simulink model "Solar_Panel_Tutorial"  (R2021b)
settings: Solver=VariableStepAuto  StartTime=0.0  StopTime=10.0  RelTol=1e-3
undefined symbols (not defined in the file): J, Kd
settings Model: Creator=mluser  LastModifiedBy=mluser

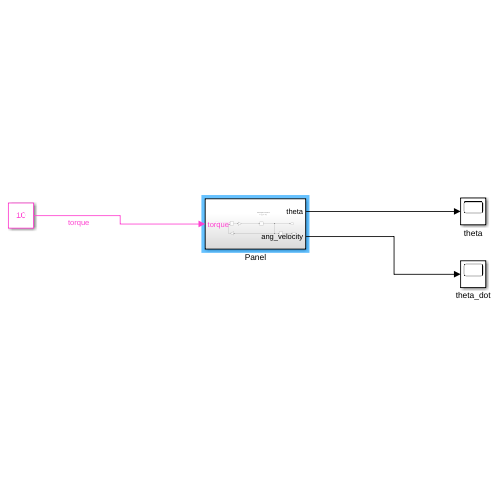
[thumbnail: Simulink's stored preview of the top-level diagram]
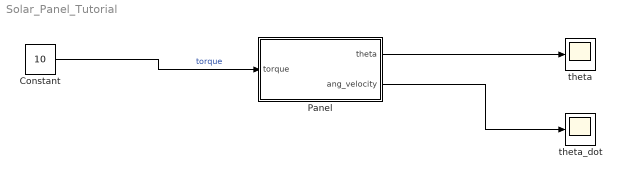
== system Solar_Panel_Tutorial ==
  Constant : Constant  Value=10
  Panel : Subsystem
  theta : Scope
  theta_dot : Scope
  wires:
  Constant/1 -> Panel/1(torque)  "torque"
  Panel/1(theta) -> theta/1
  Panel/2(ang_velocity) -> theta_dot/1

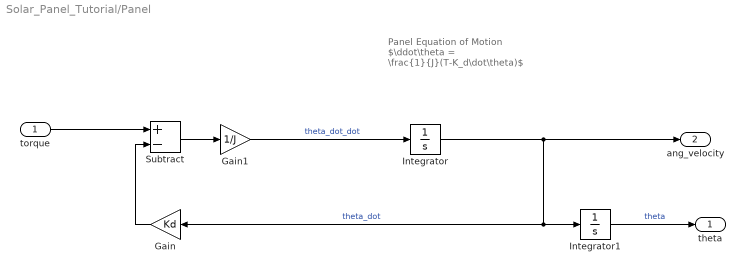
== system Solar_Panel_Tutorial/Panel ==
  note: Panel Equation of Motion
      | $\ddot\theta = \frac{1}{J}(T-K_d\dot\theta)$
  torque : Inport
  Gain : Gain  Gain=Kd
  Gain1 : Gain  Gain=1/J
  Integrator : Integrator
  Integrator1 : Integrator
  Subtract : Sum  Inputs=+-
  theta : Outport
  ang_velocity : Outport  Port=2
  wires:
  Integrator1/1 -> theta/1  "theta"
  Subtract/1 -> Gain1/1
  Gain/1 -> Subtract/2
  torque/1 -> Subtract/1
  Gain1/1 -> Integrator/1  "theta_dot_dot"
  Integrator/1 -> Gain/1, Integrator1/1, ang_velocity/1  "theta_dot"
